simulink model "x2Stage_Rocket"  (R2022b)
settings: Solver=VariableStepAuto  StartTime=0.0  StopTime=5
model workspace: external: MATLAB File C:\Users\Trenton VerKuilen\OneDrive - lmu.edu\School\Capstone\SimscapeImportFiles\x2Stage_Rocket_DataFile.m (data not in the file)
undefined symbols (not defined in the file or in its folder): F, MIL, Moderate, sigbuilder_block, smiData, X, Y, Z
libraries: sm_lib x543, nesl_utility x11, simulink_extras x3, sharedtransform x2, dspmtrx3 x2, aerolibwind2 x2, mspsensorlib x1, aerolibatmos2 x1
(part 6 of 11)

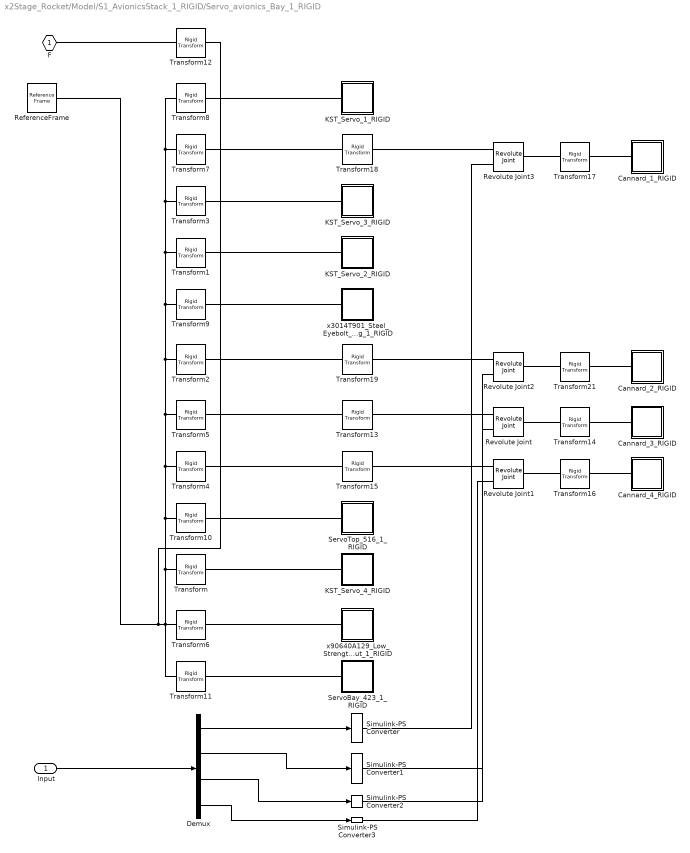
== system x2Stage_Rocket/Model/S1_AvionicsStack_1_RIGID/Servo_avionics_Bay_1_RIGID ==
  Input : Inport
  Cannard_1_RIGID : Subsystem
  Cannard_2_RIGID : Subsystem
  Cannard_3_RIGID : Subsystem
  Cannard_4_RIGID : Subsystem
  Demux : Demux
  KST_Servo_1_RIGID : Subsystem
  KST_Servo_2_RIGID : Subsystem
  KST_Servo_3_RIGID : Subsystem
  KST_Servo_4_RIGID : Subsystem
  ReferenceFrame : sm_lib/Frames and Transforms/Reference Frame
  Revolute Joint{,1..3} (4 alike) : sm_lib/Joints/Revolute Joint  JointMode=Normal  SenseConstraintForce=off  SenseConstraintForceX=off  SenseConstraintForceY=off  SenseConstraintForceZ=off  SenseConstraintTorque=off  SenseConstraintTorqueX=off  SenseConstraintTorqueY=off  SenseConstraintTorqueZ=off  SenseTotalForce=off  SenseTotalForceX=off  SenseTotalForceY=off  SenseTotalForceZ=off  SenseTotalTorque=off  SenseTotalTorqueX=off  SenseTotalTorqueY=off  SenseTotalTorqueZ=off  CompositeWrenchDir=FollowerOnBase  CompositeWrenchFrame=BaseFrame  EquilibriumPosition=0  EquilibriumPositionUnits=deg  SpringStiffness=0  SpringStiffnessUnits=N*m/deg  DampingCoefficient=0  DampingCoefficientUnits=N*m/(deg/s)  TorqueActuationMode=ComputedTorque  MotionActuationMode=InputMotion  SensePosition=off  SenseVelocity=off  SenseAcceleration=off  SenseTorqueForce=off  SenseLowerLimitTorqueForce=off  SenseUpperLimitTorqueForce=off  LowerLimitSpecify=off  LowerLimitBound=-90  LowerLimitBoundUnits=deg  LowerLimitStiffness=1e4  LowerLimitStiffnessUnits=N*m/deg  LowerLimitDamping=10  LowerLimitDampingUnits=N*m/(deg/s)  LowerLimitTransitionRegionWidth=0.1  LowerLimitTransitionRegionWidthUnits=deg  UpperLimitSpecify=off  UpperLimitBound=90  UpperLimitBoundUnits=deg  UpperLimitStiffness=1e4  UpperLimitStiffnessUnits=N*m/deg  UpperLimitDamping=10  UpperLimitDampingUnits=N*m/(deg/s)  UpperLimitTransitionRegionWidth=0.1  UpperLimitTransitionRegionWidthUnits=deg  PositionTargetSpecify=off  PositionTargetPriority=High  PositionTargetValue=0  PositionTargetValueUnits=deg  VelocityTargetSpecify=off  VelocityTargetPriority=High  VelocityTargetValue=0  VelocityTargetValueUnits=deg/s
  ServoBay_423_1_RIGID : Subsystem
  ServoTop_516_1_RIGID : Subsystem
  Simulink-PS Converter{,1..3} (4 alike) : nesl_utility/Simulink-PS Converter  PhysicalDomain=network_engine_domain  SubClassName=ps_input  LeftPortType=input  RightPortType=output  PseudoPeriodic=off  Frequencies=[]  NoiseDistribution=none  NoiseParameters=[]  Unit=1  AffineConversion=off  FilteringAndDerivatives=filter  SimscapeFilterOrder=2  InputFilterTimeConstant=0.001  UdotUserProvided=0
  Transform : sm_lib/Frames and Transforms/Rigid Transform  TranslationMethod=Cartesian  TranslationStandardOffset=0  TranslationLengthUnit=in  TranslationStandardAxis=+Z  TranslationCartesianOffset=smiData.RigidTransform(117).translation  TranslationROffset=0  TranslationROffsetUnits=m  TranslationZOffset=0  TranslationZOffsetUnits=m  TranslationThetaOffset=0  TranslationThetaOffsetUnits=deg  RotationMethod=ArbitraryAxis  RotationAngleUnits=rad  RotationStandardAxis=+Z  RotationAngle=smiData.RigidTransform(117).angle  RotationArbitraryAxis=smiData.RigidTransform(117).axis  FollAlignAxisA=+X  BaseAlignAxisA=+Y  FollAlignAxisB=+Y  BaseAlignAxisB=+Z  RotationSequenceAxes=FollowerAxes  RotationSequence=XYX  RotationSequenceAngles=[0 0 0]  RotationSequenceAnglesUnits=deg  RotationMatrix=[1 0 0; 0 1 0; 0 0 1]  Quaternion=[1 0 0 0]
  Transform1 : sm_lib/Frames and Transforms/Rigid Transform  TranslationMethod=Cartesian  TranslationStandardOffset=0  TranslationLengthUnit=in  TranslationStandardAxis=+Z  TranslationCartesianOffset=smiData.RigidTransform(118).translation  TranslationROffset=0  TranslationROffsetUnits=m  TranslationZOffset=0  TranslationZOffsetUnits=m  TranslationThetaOffset=0  TranslationThetaOffsetUnits=deg  RotationMethod=ArbitraryAxis  RotationAngleUnits=rad  RotationStandardAxis=+Z  RotationAngle=smiData.RigidTransform(118).angle  RotationArbitraryAxis=smiData.RigidTransform(118).axis  FollAlignAxisA=+X  BaseAlignAxisA=+Y  FollAlignAxisB=+Y  BaseAlignAxisB=+Z  RotationSequenceAxes=FollowerAxes  RotationSequence=XYX  RotationSequenceAngles=[0 0 0]  RotationSequenceAnglesUnits=deg  RotationMatrix=[1 0 0; 0 1 0; 0 0 1]  Quaternion=[1 0 0 0]
  Transform10 : sm_lib/Frames and Transforms/Rigid Transform  TranslationMethod=Cartesian  TranslationStandardOffset=0  TranslationLengthUnit=in  TranslationStandardAxis=+Z  TranslationCartesianOffset=smiData.RigidTransform(127).translation  TranslationROffset=0  TranslationROffsetUnits=m  TranslationZOffset=0  TranslationZOffsetUnits=m  TranslationThetaOffset=0  TranslationThetaOffsetUnits=deg  RotationMethod=ArbitraryAxis  RotationAngleUnits=rad  RotationStandardAxis=+Z  RotationAngle=smiData.RigidTransform(127).angle  RotationArbitraryAxis=smiData.RigidTransform(127).axis  FollAlignAxisA=+X  BaseAlignAxisA=+Y  FollAlignAxisB=+Y  BaseAlignAxisB=+Z  RotationSequenceAxes=FollowerAxes  RotationSequence=XYX  RotationSequenceAngles=[0 0 0]  RotationSequenceAnglesUnits=deg  RotationMatrix=[1 0 0; 0 1 0; 0 0 1]  Quaternion=[1 0 0 0]
  Transform11 : sm_lib/Frames and Transforms/Rigid Transform  TranslationMethod=Cartesian  TranslationStandardOffset=0  TranslationLengthUnit=in  TranslationStandardAxis=+Z  TranslationCartesianOffset=smiData.RigidTransform(128).translation  TranslationROffset=0  TranslationROffsetUnits=m  TranslationZOffset=0  TranslationZOffsetUnits=m  TranslationThetaOffset=0  TranslationThetaOffsetUnits=deg  RotationMethod=ArbitraryAxis  RotationAngleUnits=rad  RotationStandardAxis=+Z  RotationAngle=smiData.RigidTransform(128).angle  RotationArbitraryAxis=smiData.RigidTransform(128).axis  FollAlignAxisA=+X  BaseAlignAxisA=+Y  FollAlignAxisB=+Y  BaseAlignAxisB=+Z  RotationSequenceAxes=FollowerAxes  RotationSequence=XYX  RotationSequenceAngles=[0 0 0]  RotationSequenceAnglesUnits=deg  RotationMatrix=[1 0 0; 0 1 0; 0 0 1]  Quaternion=[1 0 0 0]
  Transform12 : sm_lib/Frames and Transforms/Rigid Transform  TranslationMethod=Cartesian  TranslationStandardOffset=0  TranslationLengthUnit=in  TranslationStandardAxis=+Z  TranslationCartesianOffset=smiData.RigidTransform(129).translation  TranslationROffset=0  TranslationROffsetUnits=m  TranslationZOffset=0  TranslationZOffsetUnits=m  TranslationThetaOffset=0  TranslationThetaOffsetUnits=deg  RotationMethod=ArbitraryAxis  RotationAngleUnits=rad  RotationStandardAxis=+Z  RotationAngle=smiData.RigidTransform(129).angle  RotationArbitraryAxis=smiData.RigidTransform(129).axis  FollAlignAxisA=+X  BaseAlignAxisA=+Y  FollAlignAxisB=+Y  BaseAlignAxisB=+Z  RotationSequenceAxes=FollowerAxes  RotationSequence=XYX  RotationSequenceAngles=[0 0 0]  RotationSequenceAnglesUnits=deg  RotationMatrix=[1 0 0; 0 1 0; 0 0 1]  Quaternion=[1 0 0 0]
  Transform{13,16..17,19} (4 alike) : sm_lib/Frames and Transforms/Rigid Transform  TranslationMethod=None  TranslationStandardOffset=0  TranslationLengthUnit=in  TranslationStandardAxis=+Z  TranslationCartesianOffset=smiData.RigidTransform(114).translation  TranslationROffset=0  TranslationROffsetUnits=m  TranslationZOffset=0  TranslationZOffsetUnits=m  TranslationThetaOffset=0  TranslationThetaOffsetUnits=deg  RotationMethod=StandardAxis  RotationAngleUnits=deg  RotationStandardAxis=+Y  RotationAngle=-90  RotationArbitraryAxis=smiData.RigidTransform(114).axis  FollAlignAxisA=+X  BaseAlignAxisA=+Y  FollAlignAxisB=+Y  BaseAlignAxisB=+Z  RotationSequenceAxes=FollowerAxes  RotationSequence=XYX  RotationSequenceAngles=[0 0 0]  RotationSequenceAnglesUnits=deg  RotationMatrix=[1 0 0; 0 1 0; 0 0 1]  Quaternion=[1 0 0 0]
  Transform{14..15,18,21} (4 alike) : sm_lib/Frames and Transforms/Rigid Transform  TranslationMethod=None  TranslationStandardOffset=0  TranslationLengthUnit=in  TranslationStandardAxis=+Z  TranslationCartesianOffset=smiData.RigidTransform(114).translation  TranslationROffset=0  TranslationROffsetUnits=m  TranslationZOffset=0  TranslationZOffsetUnits=m  TranslationThetaOffset=0  TranslationThetaOffsetUnits=deg  RotationMethod=StandardAxis  RotationAngleUnits=deg  RotationStandardAxis=+Y  RotationAngle=90  RotationArbitraryAxis=smiData.RigidTransform(114).axis  FollAlignAxisA=+X  BaseAlignAxisA=+Y  FollAlignAxisB=+Y  BaseAlignAxisB=+Z  RotationSequenceAxes=FollowerAxes  RotationSequence=XYX  RotationSequenceAngles=[0 0 0]  RotationSequenceAnglesUnits=deg  RotationMatrix=[1 0 0; 0 1 0; 0 0 1]  Quaternion=[1 0 0 0]
  Transform2 : sm_lib/Frames and Transforms/Rigid Transform  TranslationMethod=Cartesian  TranslationStandardOffset=0  TranslationLengthUnit=in  TranslationStandardAxis=+Z  TranslationCartesianOffset=smiData.RigidTransform(119).translation  TranslationROffset=0  TranslationROffsetUnits=m  TranslationZOffset=0  TranslationZOffsetUnits=m  TranslationThetaOffset=0  TranslationThetaOffsetUnits=deg  RotationMethod=ArbitraryAxis  RotationAngleUnits=rad  RotationStandardAxis=+Z  RotationAngle=smiData.RigidTransform(119).angle  RotationArbitraryAxis=smiData.RigidTransform(119).axis  FollAlignAxisA=+X  BaseAlignAxisA=+Y  FollAlignAxisB=+Y  BaseAlignAxisB=+Z  RotationSequenceAxes=FollowerAxes  RotationSequence=XYX  RotationSequenceAngles=[0 0 0]  RotationSequenceAnglesUnits=deg  RotationMatrix=[1 0 0; 0 1 0; 0 0 1]  Quaternion=[1 0 0 0]
  Transform3 : sm_lib/Frames and Transforms/Rigid Transform  TranslationMethod=Cartesian  TranslationStandardOffset=0  TranslationLengthUnit=in  TranslationStandardAxis=+Z  TranslationCartesianOffset=smiData.RigidTransform(120).translation  TranslationROffset=0  TranslationROffsetUnits=m  TranslationZOffset=0  TranslationZOffsetUnits=m  TranslationThetaOffset=0  TranslationThetaOffsetUnits=deg  RotationMethod=ArbitraryAxis  RotationAngleUnits=rad  RotationStandardAxis=+Z  RotationAngle=smiData.RigidTransform(120).angle  RotationArbitraryAxis=smiData.RigidTransform(120).axis  FollAlignAxisA=+X  BaseAlignAxisA=+Y  FollAlignAxisB=+Y  BaseAlignAxisB=+Z  RotationSequenceAxes=FollowerAxes  RotationSequence=XYX  RotationSequenceAngles=[0 0 0]  RotationSequenceAnglesUnits=deg  RotationMatrix=[1 0 0; 0 1 0; 0 0 1]  Quaternion=[1 0 0 0]
  Transform4 : sm_lib/Frames and Transforms/Rigid Transform  TranslationMethod=Cartesian  TranslationStandardOffset=0  TranslationLengthUnit=in  TranslationStandardAxis=+Z  TranslationCartesianOffset=smiData.RigidTransform(121).translation  TranslationROffset=0  TranslationROffsetUnits=m  TranslationZOffset=0  TranslationZOffsetUnits=m  TranslationThetaOffset=0  TranslationThetaOffsetUnits=deg  RotationMethod=ArbitraryAxis  RotationAngleUnits=rad  RotationStandardAxis=+Z  RotationAngle=smiData.RigidTransform(121).angle  RotationArbitraryAxis=smiData.RigidTransform(121).axis  FollAlignAxisA=+X  BaseAlignAxisA=+Y  FollAlignAxisB=+Y  BaseAlignAxisB=+Z  RotationSequenceAxes=FollowerAxes  RotationSequence=XYX  RotationSequenceAngles=[0 0 0]  RotationSequenceAnglesUnits=deg  RotationMatrix=[1 0 0; 0 1 0; 0 0 1]  Quaternion=[1 0 0 0]
  Transform5 : sm_lib/Frames and Transforms/Rigid Transform  TranslationMethod=Cartesian  TranslationStandardOffset=0  TranslationLengthUnit=in  TranslationStandardAxis=+Z  TranslationCartesianOffset=smiData.RigidTransform(122).translation  TranslationROffset=0  TranslationROffsetUnits=m  TranslationZOffset=0  TranslationZOffsetUnits=m  TranslationThetaOffset=0  TranslationThetaOffsetUnits=deg  RotationMethod=ArbitraryAxis  RotationAngleUnits=rad  RotationStandardAxis=+Z  RotationAngle=smiData.RigidTransform(122).angle  RotationArbitraryAxis=smiData.RigidTransform(122).axis  FollAlignAxisA=+X  BaseAlignAxisA=+Y  FollAlignAxisB=+Y  BaseAlignAxisB=+Z  RotationSequenceAxes=FollowerAxes  RotationSequence=XYX  RotationSequenceAngles=[0 0 0]  RotationSequenceAnglesUnits=deg  RotationMatrix=[1 0 0; 0 1 0; 0 0 1]  Quaternion=[1 0 0 0]
  Transform6 : sm_lib/Frames and Transforms/Rigid Transform  TranslationMethod=Cartesian  TranslationStandardOffset=0  TranslationLengthUnit=in  TranslationStandardAxis=+Z  TranslationCartesianOffset=smiData.RigidTransform(123).translation  TranslationROffset=0  TranslationROffsetUnits=m  TranslationZOffset=0  TranslationZOffsetUnits=m  TranslationThetaOffset=0  TranslationThetaOffsetUnits=deg  RotationMethod=ArbitraryAxis  RotationAngleUnits=rad  RotationStandardAxis=+Z  RotationAngle=smiData.RigidTransform(123).angle  RotationArbitraryAxis=smiData.RigidTransform(123).axis  FollAlignAxisA=+X  BaseAlignAxisA=+Y  FollAlignAxisB=+Y  BaseAlignAxisB=+Z  RotationSequenceAxes=FollowerAxes  RotationSequence=XYX  RotationSequenceAngles=[0 0 0]  RotationSequenceAnglesUnits=deg  RotationMatrix=[1 0 0; 0 1 0; 0 0 1]  Quaternion=[1 0 0 0]
  Transform7 : sm_lib/Frames and Transforms/Rigid Transform  TranslationMethod=Cartesian  TranslationStandardOffset=0  TranslationLengthUnit=in  TranslationStandardAxis=+Z  TranslationCartesianOffset=smiData.RigidTransform(124).translation  TranslationROffset=0  TranslationROffsetUnits=m  TranslationZOffset=0  TranslationZOffsetUnits=m  TranslationThetaOffset=0  TranslationThetaOffsetUnits=deg  RotationMethod=ArbitraryAxis  RotationAngleUnits=rad  RotationStandardAxis=+Z  RotationAngle=smiData.RigidTransform(124).angle  RotationArbitraryAxis=smiData.RigidTransform(124).axis  FollAlignAxisA=+X  BaseAlignAxisA=+Y  FollAlignAxisB=+Y  BaseAlignAxisB=+Z  RotationSequenceAxes=FollowerAxes  RotationSequence=XYX  RotationSequenceAngles=[0 0 0]  RotationSequenceAnglesUnits=deg  RotationMatrix=[1 0 0; 0 1 0; 0 0 1]  Quaternion=[1 0 0 0]
  Transform8 : sm_lib/Frames and Transforms/Rigid Transform  TranslationMethod=Cartesian  TranslationStandardOffset=0  TranslationLengthUnit=in  TranslationStandardAxis=+Z  TranslationCartesianOffset=smiData.RigidTransform(125).translation  TranslationROffset=0  TranslationROffsetUnits=m  TranslationZOffset=0  TranslationZOffsetUnits=m  TranslationThetaOffset=0  TranslationThetaOffsetUnits=deg  RotationMethod=ArbitraryAxis  RotationAngleUnits=rad  RotationStandardAxis=+Z  RotationAngle=smiData.RigidTransform(125).angle  RotationArbitraryAxis=smiData.RigidTransform(125).axis  FollAlignAxisA=+X  BaseAlignAxisA=+Y  FollAlignAxisB=+Y  BaseAlignAxisB=+Z  RotationSequenceAxes=FollowerAxes  RotationSequence=XYX  RotationSequenceAngles=[0 0 0]  RotationSequenceAnglesUnits=deg  RotationMatrix=[1 0 0; 0 1 0; 0 0 1]  Quaternion=[1 0 0 0]
  Transform9 : sm_lib/Frames and Transforms/Rigid Transform  TranslationMethod=Cartesian  TranslationStandardOffset=0  TranslationLengthUnit=in  TranslationStandardAxis=+Z  TranslationCartesianOffset=smiData.RigidTransform(126).translation  TranslationROffset=0  TranslationROffsetUnits=m  TranslationZOffset=0  TranslationZOffsetUnits=m  TranslationThetaOffset=0  TranslationThetaOffsetUnits=deg  RotationMethod=ArbitraryAxis  RotationAngleUnits=rad  RotationStandardAxis=+Z  RotationAngle=smiData.RigidTransform(126).angle  RotationArbitraryAxis=smiData.RigidTransform(126).axis  FollAlignAxisA=+X  BaseAlignAxisA=+Y  FollAlignAxisB=+Y  BaseAlignAxisB=+Z  RotationSequenceAxes=FollowerAxes  RotationSequence=XYX  RotationSequenceAngles=[0 0 0]  RotationSequenceAnglesUnits=deg  RotationMatrix=[1 0 0; 0 1 0; 0 0 1]  Quaternion=[1 0 0 0]
  x3014T901_Steel_Eyebolt_with_Shoulder_for_Lifting_1_RIGID : Subsystem
  x90640A129_Low_Strength_Steel_Nylon_Insert_Locknut_1_RIGID : Subsystem
  F : PMIOPort  Side=Right
  wires:
  Input/1 -> Demux/1
  Demux/1 -> Simulink-PS Converter/1
  Demux/2 -> Simulink-PS Converter1/1
  Demux/3 -> Simulink-PS Converter2/1
  Demux/4 -> Simulink-PS Converter3/1
  connections:
  F/RConn1 -- Transform12/LConn1
  Revolute Joint1/RConn1 -- Transform16/LConn1
  Transform8/RConn1 -- KST_Servo_1_RIGID/LConn1
  Revolute Joint3/RConn1 -- Transform17/LConn1
  ReferenceFrame/RConn1 -- Transform7/LConn1 -- Transform8/LConn1 -- Transform3/LConn1 -- Transform1/LConn1 -- Transform9/LConn1 -- Transform2/LConn1 -- Transform5/LConn1 -- Transform4/LConn1 -- Transform10/LConn1 -- Transform/LConn1 -- Transform6/LConn1 -- Transform11/LConn1 -- Transform12/RConn1
  Transform3/RConn1 -- KST_Servo_3_RIGID/LConn1
  Transform7/RConn1 -- Transform18/LConn1
  Transform1/RConn1 -- KST_Servo_2_RIGID/LConn1
  Transform9/RConn1 -- x3014T901_Steel_Eyebolt_with_Shoulder_for_Lifting_1_RIGID/LConn1
  Transform2/RConn1 -- Transform19/LConn1
  Transform5/RConn1 -- Transform13/LConn1
  Transform4/RConn1 -- Transform15/LConn1
  Transform10/RConn1 -- ServoTop_516_1_RIGID/LConn1
  Transform/RConn1 -- KST_Servo_4_RIGID/LConn1
  Transform6/RConn1 -- x90640A129_Low_Strength_Steel_Nylon_Insert_Locknut_1_RIGID/LConn1
  Transform11/RConn1 -- ServoBay_423_1_RIGID/LConn1
  Transform19/RConn1 -- Revolute Joint2/LConn1
  Transform18/RConn1 -- Revolute Joint3/LConn1
  Transform13/RConn1 -- Revolute Joint/LConn1
  Transform15/RConn1 -- Revolute Joint1/LConn1
  Simulink-PS Converter/RConn1 -- Revolute Joint3/LConn2
  Simulink-PS Converter1/RConn1 -- Revolute Joint2/LConn2
  Simulink-PS Converter2/RConn1 -- Revolute Joint/LConn2
  Simulink-PS Converter3/RConn1 -- Revolute Joint1/LConn2
  Revolute Joint2/RConn1 -- Transform21/LConn1
  Revolute Joint/RConn1 -- Transform14/LConn1
  Transform17/RConn1 -- Cannard_1_RIGID/LConn1
  Transform21/RConn1 -- Cannard_2_RIGID/LConn1
  Transform14/RConn1 -- Cannard_3_RIGID/LConn1
  Transform16/RConn1 -- Cannard_4_RIGID/LConn1

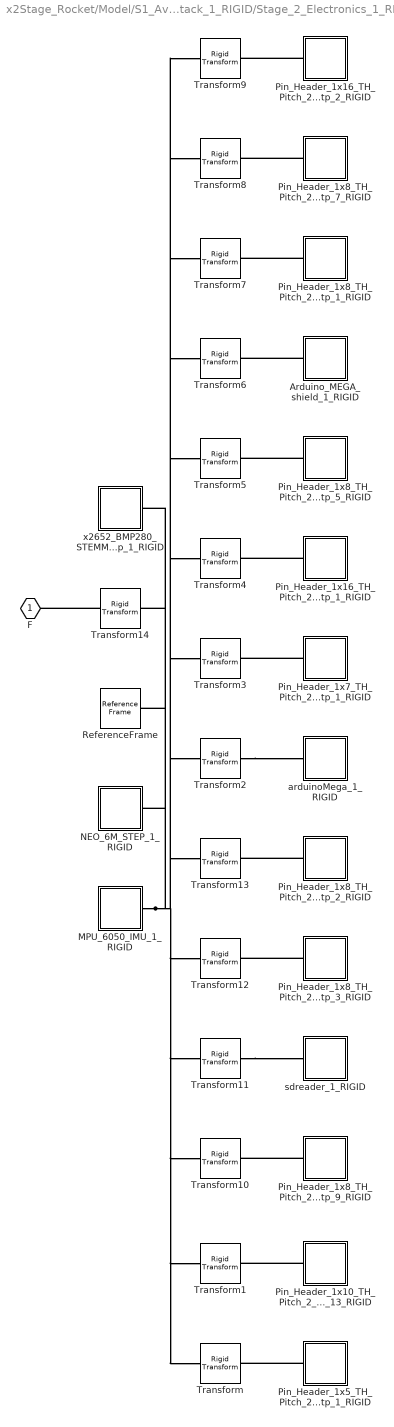
== system x2Stage_Rocket/Model/S1_AvionicsStack_1_RIGID/Stage_2_Electronics_1_RIGID ==
  Arduino_MEGA_shield_1_RIGID : Subsystem
  MPU_6050_IMU_1_RIGID : Subsystem
  NEO_6M_STEP_1_RIGID : Subsystem
  Pin_Header_1x10_TH_Pitch_2_54mm_stp_13_RIGID : Subsystem
  Pin_Header_1x16_TH_Pitch_2_54mm_stp_1_RIGID : Subsystem
  Pin_Header_1x16_TH_Pitch_2_54mm_stp_2_RIGID : Subsystem
  Pin_Header_1x5_TH_Pitch_2_54mm_stp_1_RIGID : Subsystem
  Pin_Header_1x7_TH_Pitch_2_54mm_stp_1_RIGID : Subsystem
  Pin_Header_1x8_TH_Pitch_2_54mm_stp_1_RIGID : Subsystem
  Pin_Header_1x8_TH_Pitch_2_54mm_stp_2_RIGID : Subsystem
  Pin_Header_1x8_TH_Pitch_2_54mm_stp_3_RIGID : Subsystem
  Pin_Header_1x8_TH_Pitch_2_54mm_stp_5_RIGID : Subsystem
  Pin_Header_1x8_TH_Pitch_2_54mm_stp_7_RIGID : Subsystem
  Pin_Header_1x8_TH_Pitch_2_54mm_stp_9_RIGID : Subsystem
  ReferenceFrame : sm_lib/Frames and Transforms/Reference Frame
  Transform : sm_lib/Frames and Transforms/Rigid Transform  TranslationMethod=Cartesian  TranslationStandardOffset=0  TranslationLengthUnit=in  TranslationStandardAxis=+Z  TranslationCartesianOffset=smiData.RigidTransform(77).translation  TranslationROffset=0  TranslationROffsetUnits=m  TranslationZOffset=0  TranslationZOffsetUnits=m  TranslationThetaOffset=0  TranslationThetaOffsetUnits=deg  RotationMethod=ArbitraryAxis  RotationAngleUnits=rad  RotationStandardAxis=+Z  RotationAngle=smiData.RigidTransform(77).angle  RotationArbitraryAxis=smiData.RigidTransform(77).axis  FollAlignAxisA=+X  BaseAlignAxisA=+Y  FollAlignAxisB=+Y  BaseAlignAxisB=+Z  RotationSequenceAxes=FollowerAxes  RotationSequence=XYX  RotationSequenceAngles=[0 0 0]  RotationSequenceAnglesUnits=deg  RotationMatrix=[1 0 0; 0 1 0; 0 0 1]  Quaternion=[1 0 0 0]
  Transform1 : sm_lib/Frames and Transforms/Rigid Transform  TranslationMethod=Cartesian  TranslationStandardOffset=0  TranslationLengthUnit=in  TranslationStandardAxis=+Z  TranslationCartesianOffset=smiData.RigidTransform(78).translation  TranslationROffset=0  TranslationROffsetUnits=m  TranslationZOffset=0  TranslationZOffsetUnits=m  TranslationThetaOffset=0  TranslationThetaOffsetUnits=deg  RotationMethod=ArbitraryAxis  RotationAngleUnits=rad  RotationStandardAxis=+Z  RotationAngle=smiData.RigidTransform(78).angle  RotationArbitraryAxis=smiData.RigidTransform(78).axis  FollAlignAxisA=+X  BaseAlignAxisA=+Y  FollAlignAxisB=+Y  BaseAlignAxisB=+Z  RotationSequenceAxes=FollowerAxes  RotationSequence=XYX  RotationSequenceAngles=[0 0 0]  RotationSequenceAnglesUnits=deg  RotationMatrix=[1 0 0; 0 1 0; 0 0 1]  Quaternion=[1 0 0 0]
  Transform10 : sm_lib/Frames and Transforms/Rigid Transform  TranslationMethod=Cartesian  TranslationStandardOffset=0  TranslationLengthUnit=in  TranslationStandardAxis=+Z  TranslationCartesianOffset=smiData.RigidTransform(87).translation  TranslationROffset=0  TranslationROffsetUnits=m  TranslationZOffset=0  TranslationZOffsetUnits=m  TranslationThetaOffset=0  TranslationThetaOffsetUnits=deg  RotationMethod=ArbitraryAxis  RotationAngleUnits=rad  RotationStandardAxis=+Z  RotationAngle=smiData.RigidTransform(87).angle  RotationArbitraryAxis=smiData.RigidTransform(87).axis  FollAlignAxisA=+X  BaseAlignAxisA=+Y  FollAlignAxisB=+Y  BaseAlignAxisB=+Z  RotationSequenceAxes=FollowerAxes  RotationSequence=XYX  RotationSequenceAngles=[0 0 0]  RotationSequenceAnglesUnits=deg  RotationMatrix=[1 0 0; 0 1 0; 0 0 1]  Quaternion=[1 0 0 0]
  Transform11 : sm_lib/Frames and Transforms/Rigid Transform  TranslationMethod=Cartesian  TranslationStandardOffset=0  TranslationLengthUnit=in  TranslationStandardAxis=+Z  TranslationCartesianOffset=smiData.RigidTransform(88).translation  TranslationROffset=0  TranslationROffsetUnits=m  TranslationZOffset=0  TranslationZOffsetUnits=m  TranslationThetaOffset=0  TranslationThetaOffsetUnits=deg  RotationMethod=ArbitraryAxis  RotationAngleUnits=rad  RotationStandardAxis=+Z  RotationAngle=smiData.RigidTransform(88).angle  RotationArbitraryAxis=smiData.RigidTransform(88).axis  FollAlignAxisA=+X  BaseAlignAxisA=+Y  FollAlignAxisB=+Y  BaseAlignAxisB=+Z  RotationSequenceAxes=FollowerAxes  RotationSequence=XYX  RotationSequenceAngles=[0 0 0]  RotationSequenceAnglesUnits=deg  RotationMatrix=[1 0 0; 0 1 0; 0 0 1]  Quaternion=[1 0 0 0]
  Transform12 : sm_lib/Frames and Transforms/Rigid Transform  TranslationMethod=Cartesian  TranslationStandardOffset=0  TranslationLengthUnit=in  TranslationStandardAxis=+Z  TranslationCartesianOffset=smiData.RigidTransform(89).translation  TranslationROffset=0  TranslationROffsetUnits=m  TranslationZOffset=0  TranslationZOffsetUnits=m  TranslationThetaOffset=0  TranslationThetaOffsetUnits=deg  RotationMethod=ArbitraryAxis  RotationAngleUnits=rad  RotationStandardAxis=+Z  RotationAngle=smiData.RigidTransform(89).angle  RotationArbitraryAxis=smiData.RigidTransform(89).axis  FollAlignAxisA=+X  BaseAlignAxisA=+Y  FollAlignAxisB=+Y  BaseAlignAxisB=+Z  RotationSequenceAxes=FollowerAxes  RotationSequence=XYX  RotationSequenceAngles=[0 0 0]  RotationSequenceAnglesUnits=deg  RotationMatrix=[1 0 0; 0 1 0; 0 0 1]  Quaternion=[1 0 0 0]
  Transform13 : sm_lib/Frames and Transforms/Rigid Transform  TranslationMethod=Cartesian  TranslationStandardOffset=0  TranslationLengthUnit=in  TranslationStandardAxis=+Z  TranslationCartesianOffset=smiData.RigidTransform(106).translation  TranslationROffset=0  TranslationROffsetUnits=m  TranslationZOffset=0  TranslationZOffsetUnits=m  TranslationThetaOffset=0  TranslationThetaOffsetUnits=deg  RotationMethod=ArbitraryAxis  RotationAngleUnits=rad  RotationStandardAxis=+Z  RotationAngle=smiData.RigidTransform(106).angle  RotationArbitraryAxis=smiData.RigidTransform(106).axis  FollAlignAxisA=+X  BaseAlignAxisA=+Y  FollAlignAxisB=+Y  BaseAlignAxisB=+Z  RotationSequenceAxes=FollowerAxes  RotationSequence=XYX  RotationSequenceAngles=[0 0 0]  RotationSequenceAnglesUnits=deg  RotationMatrix=[1 0 0; 0 1 0; 0 0 1]  Quaternion=[1 0 0 0]
  Transform14 : sm_lib/Frames and Transforms/Rigid Transform  TranslationMethod=Cartesian  TranslationStandardOffset=0  TranslationLengthUnit=in  TranslationStandardAxis=+Z  TranslationCartesianOffset=smiData.RigidTransform(111).translation  TranslationROffset=0  TranslationROffsetUnits=m  TranslationZOffset=0  TranslationZOffsetUnits=m  TranslationThetaOffset=0  TranslationThetaOffsetUnits=deg  RotationMethod=ArbitraryAxis  RotationAngleUnits=rad  RotationStandardAxis=+Z  RotationAngle=smiData.RigidTransform(111).angle  RotationArbitraryAxis=smiData.RigidTransform(111).axis  FollAlignAxisA=+X  BaseAlignAxisA=+Y  FollAlignAxisB=+Y  BaseAlignAxisB=+Z  RotationSequenceAxes=FollowerAxes  RotationSequence=XYX  RotationSequenceAngles=[0 0 0]  RotationSequenceAnglesUnits=deg  RotationMatrix=[1 0 0; 0 1 0; 0 0 1]  Quaternion=[1 0 0 0]
  Transform2 : sm_lib/Frames and Transforms/Rigid Transform  TranslationMethod=Cartesian  TranslationStandardOffset=0  TranslationLengthUnit=in  TranslationStandardAxis=+Z  TranslationCartesianOffset=smiData.RigidTransform(79).translation  TranslationROffset=0  TranslationROffsetUnits=m  TranslationZOffset=0  TranslationZOffsetUnits=m  TranslationThetaOffset=0  TranslationThetaOffsetUnits=deg  RotationMethod=ArbitraryAxis  RotationAngleUnits=rad  RotationStandardAxis=+Z  RotationAngle=smiData.RigidTransform(79).angle  RotationArbitraryAxis=smiData.RigidTransform(79).axis  FollAlignAxisA=+X  BaseAlignAxisA=+Y  FollAlignAxisB=+Y  BaseAlignAxisB=+Z  RotationSequenceAxes=FollowerAxes  RotationSequence=XYX  RotationSequenceAngles=[0 0 0]  RotationSequenceAnglesUnits=deg  RotationMatrix=[1 0 0; 0 1 0; 0 0 1]  Quaternion=[1 0 0 0]
  Transform3 : sm_lib/Frames and Transforms/Rigid Transform  TranslationMethod=Cartesian  TranslationStandardOffset=0  TranslationLengthUnit=in  TranslationStandardAxis=+Z  TranslationCartesianOffset=smiData.RigidTransform(80).translation  TranslationROffset=0  TranslationROffsetUnits=m  TranslationZOffset=0  TranslationZOffsetUnits=m  TranslationThetaOffset=0  TranslationThetaOffsetUnits=deg  RotationMethod=ArbitraryAxis  RotationAngleUnits=rad  RotationStandardAxis=+Z  RotationAngle=smiData.RigidTransform(80).angle  RotationArbitraryAxis=smiData.RigidTransform(80).axis  FollAlignAxisA=+X  BaseAlignAxisA=+Y  FollAlignAxisB=+Y  BaseAlignAxisB=+Z  RotationSequenceAxes=FollowerAxes  RotationSequence=XYX  RotationSequenceAngles=[0 0 0]  RotationSequenceAnglesUnits=deg  RotationMatrix=[1 0 0; 0 1 0; 0 0 1]  Quaternion=[1 0 0 0]
  Transform4 : sm_lib/Frames and Transforms/Rigid Transform  TranslationMethod=Cartesian  TranslationStandardOffset=0  TranslationLengthUnit=in  TranslationStandardAxis=+Z  TranslationCartesianOffset=smiData.RigidTransform(81).translation  TranslationROffset=0  TranslationROffsetUnits=m  TranslationZOffset=0  TranslationZOffsetUnits=m  TranslationThetaOffset=0  TranslationThetaOffsetUnits=deg  RotationMethod=ArbitraryAxis  RotationAngleUnits=rad  RotationStandardAxis=+Z  RotationAngle=smiData.RigidTransform(81).angle  RotationArbitraryAxis=smiData.RigidTransform(81).axis  FollAlignAxisA=+X  BaseAlignAxisA=+Y  FollAlignAxisB=+Y  BaseAlignAxisB=+Z  RotationSequenceAxes=FollowerAxes  RotationSequence=XYX  RotationSequenceAngles=[0 0 0]  RotationSequenceAnglesUnits=deg  RotationMatrix=[1 0 0; 0 1 0; 0 0 1]  Quaternion=[1 0 0 0]
  Transform5 : sm_lib/Frames and Transforms/Rigid Transform  TranslationMethod=Cartesian  TranslationStandardOffset=0  TranslationLengthUnit=in  TranslationStandardAxis=+Z  TranslationCartesianOffset=smiData.RigidTransform(82).translation  TranslationROffset=0  TranslationROffsetUnits=m  TranslationZOffset=0  TranslationZOffsetUnits=m  TranslationThetaOffset=0  TranslationThetaOffsetUnits=deg  RotationMethod=ArbitraryAxis  RotationAngleUnits=rad  RotationStandardAxis=+Z  RotationAngle=smiData.RigidTransform(82).angle  RotationArbitraryAxis=smiData.RigidTransform(82).axis  FollAlignAxisA=+X  BaseAlignAxisA=+Y  FollAlignAxisB=+Y  BaseAlignAxisB=+Z  RotationSequenceAxes=FollowerAxes  RotationSequence=XYX  RotationSequenceAngles=[0 0 0]  RotationSequenceAnglesUnits=deg  RotationMatrix=[1 0 0; 0 1 0; 0 0 1]  Quaternion=[1 0 0 0]
  Transform6 : sm_lib/Frames and Transforms/Rigid Transform  TranslationMethod=Cartesian  TranslationStandardOffset=0  TranslationLengthUnit=in  TranslationStandardAxis=+Z  TranslationCartesianOffset=smiData.RigidTransform(83).translation  TranslationROffset=0  TranslationROffsetUnits=m  TranslationZOffset=0  TranslationZOffsetUnits=m  TranslationThetaOffset=0  TranslationThetaOffsetUnits=deg  RotationMethod=ArbitraryAxis  RotationAngleUnits=rad  RotationStandardAxis=+Z  RotationAngle=smiData.RigidTransform(83).angle  RotationArbitraryAxis=smiData.RigidTransform(83).axis  FollAlignAxisA=+X  BaseAlignAxisA=+Y  FollAlignAxisB=+Y  BaseAlignAxisB=+Z  RotationSequenceAxes=FollowerAxes  RotationSequence=XYX  RotationSequenceAngles=[0 0 0]  RotationSequenceAnglesUnits=deg  RotationMatrix=[1 0 0; 0 1 0; 0 0 1]  Quaternion=[1 0 0 0]
  Transform7 : sm_lib/Frames and Transforms/Rigid Transform  TranslationMethod=Cartesian  TranslationStandardOffset=0  TranslationLengthUnit=in  TranslationStandardAxis=+Z  TranslationCartesianOffset=smiData.RigidTransform(84).translation  TranslationROffset=0  TranslationROffsetUnits=m  TranslationZOffset=0  TranslationZOffsetUnits=m  TranslationThetaOffset=0  TranslationThetaOffsetUnits=deg  RotationMethod=ArbitraryAxis  RotationAngleUnits=rad  RotationStandardAxis=+Z  RotationAngle=smiData.RigidTransform(84).angle  RotationArbitraryAxis=smiData.RigidTransform(84).axis  FollAlignAxisA=+X  BaseAlignAxisA=+Y  FollAlignAxisB=+Y  BaseAlignAxisB=+Z  RotationSequenceAxes=FollowerAxes  RotationSequence=XYX  RotationSequenceAngles=[0 0 0]  RotationSequenceAnglesUnits=deg  RotationMatrix=[1 0 0; 0 1 0; 0 0 1]  Quaternion=[1 0 0 0]
  Transform8 : sm_lib/Frames and Transforms/Rigid Transform  TranslationMethod=Cartesian  TranslationStandardOffset=0  TranslationLengthUnit=in  TranslationStandardAxis=+Z  TranslationCartesianOffset=smiData.RigidTransform(85).translation  TranslationROffset=0  TranslationROffsetUnits=m  TranslationZOffset=0  TranslationZOffsetUnits=m  TranslationThetaOffset=0  TranslationThetaOffsetUnits=deg  RotationMethod=ArbitraryAxis  RotationAngleUnits=rad  RotationStandardAxis=+Z  RotationAngle=smiData.RigidTransform(85).angle  RotationArbitraryAxis=smiData.RigidTransform(85).axis  FollAlignAxisA=+X  BaseAlignAxisA=+Y  FollAlignAxisB=+Y  BaseAlignAxisB=+Z  RotationSequenceAxes=FollowerAxes  RotationSequence=XYX  RotationSequenceAngles=[0 0 0]  RotationSequenceAnglesUnits=deg  RotationMatrix=[1 0 0; 0 1 0; 0 0 1]  Quaternion=[1 0 0 0]
  Transform9 : sm_lib/Frames and Transforms/Rigid Transform  TranslationMethod=Cartesian  TranslationStandardOffset=0  TranslationLengthUnit=in  TranslationStandardAxis=+Z  TranslationCartesianOffset=smiData.RigidTransform(86).translation  TranslationROffset=0  TranslationROffsetUnits=m  TranslationZOffset=0  TranslationZOffsetUnits=m  TranslationThetaOffset=0  TranslationThetaOffsetUnits=deg  RotationMethod=ArbitraryAxis  RotationAngleUnits=rad  RotationStandardAxis=+Z  RotationAngle=smiData.RigidTransform(86).angle  RotationArbitraryAxis=smiData.RigidTransform(86).axis  FollAlignAxisA=+X  BaseAlignAxisA=+Y  FollAlignAxisB=+Y  BaseAlignAxisB=+Z  RotationSequenceAxes=FollowerAxes  RotationSequence=XYX  RotationSequenceAngles=[0 0 0]  RotationSequenceAnglesUnits=deg  RotationMatrix=[1 0 0; 0 1 0; 0 0 1]  Quaternion=[1 0 0 0]
  arduinoMega_1_RIGID : Subsystem
  sdreader_1_RIGID : Subsystem
  x2652_BMP280_STEMMA_QT_step_1_RIGID : Subsystem
  F : PMIOPort  Side=Right
  connections:
  Pin_Header_1x5_TH_Pitch_2_54mm_stp_1_RIGID/LConn1 -- Transform/RConn1
  Pin_Header_1x10_TH_Pitch_2_54mm_stp_13_RIGID/LConn1 -- Transform1/RConn1
  Pin_Header_1x8_TH_Pitch_2_54mm_stp_9_RIGID/LConn1 -- Transform10/RConn1
  Transform11/RConn1 -- sdreader_1_RIGID/LConn1
  Pin_Header_1x8_TH_Pitch_2_54mm_stp_3_RIGID/LConn1 -- Transform12/RConn1
  Pin_Header_1x8_TH_Pitch_2_54mm_stp_2_RIGID/LConn1 -- Transform13/RConn1
  MPU_6050_IMU_1_RIGID/RConn1 -- NEO_6M_STEP_1_RIGID/RConn1 -- ReferenceFrame/RConn1 -- Transform/LConn1 -- Transform1/LConn1 -- Transform10/LConn1 -- Transform11/LConn1 -- Transform12/LConn1 -- Transform13/LConn1 -- Transform14/RConn1 -- Transform2/LConn1 -- Transform3/LConn1 -- Transform4/LConn1 -- Transform5/LConn1 -- Transform6/LConn1 -- Transform7/LConn1 -- Transform8/LConn1 -- Transform9/LConn1 -- x2652_BMP280_STEMMA_QT_step_1_RIGID/RConn1
  Transform14/LConn1 -- F/RConn1
  Transform2/RConn1 -- arduinoMega_1_RIGID/LConn1
  Pin_Header_1x7_TH_Pitch_2_54mm_stp_1_RIGID/LConn1 -- Transform3/RConn1
  Pin_Header_1x16_TH_Pitch_2_54mm_stp_1_RIGID/LConn1 -- Transform4/RConn1
  Pin_Header_1x8_TH_Pitch_2_54mm_stp_5_RIGID/LConn1 -- Transform5/RConn1
  Arduino_MEGA_shield_1_RIGID/LConn1 -- Transform6/RConn1
  Pin_Header_1x8_TH_Pitch_2_54mm_stp_1_RIGID/LConn1 -- Transform7/RConn1
  Pin_Header_1x8_TH_Pitch_2_54mm_stp_7_RIGID/LConn1 -- Transform8/RConn1
  Pin_Header_1x16_TH_Pitch_2_54mm_stp_2_RIGID/LConn1 -- Transform9/RConn1

== system x2Stage_Rocket/Model/S1_AvionicsStack_1_RIGID/StagingCoupler_1_RIGID ==
  ReferenceFrame : sm_lib/Frames and Transforms/Reference Frame
  Solid : sm_lib/Body Elements/File Solid  ExtGeomFileName=StagingCoupler_Default_sldprt.STEP  UnitType=FromFile  ExtGeomFileUnits=m  StepReaderType=HEX  ExportConvexHullGeometry=off  InertiaType=Custom  Mass=smiData.Solid(41).mass  MassUnits=kg  CenterOfMass=smiData.Solid(41).CoM  CenterOfMassUnits=cm  MomentsOfInertia=smiData.Solid(41).MoI  MomentsOfInertiaUnits=kg*cm^2  ProductsOfInertia=smiData.Solid(41).PoI  ProductsOfInertiaUnits=kg*cm^2  BasedOnType=DensityFromFile  Density=1000  DensityUnits=kg/m^3  DoExposeReferenceFrame=on  SerializedFrames=<Frames/>  GraphicType=FromGeometry  MarkerShape=Sphere  MarkerSize=10  GraphicVisPropType=SimpleVisualProperties  GraphicDiffuseColor=smiData.Solid(41).color  GraphicSpecularColor=[0.5 0.5 0.5 1.0]  GraphicAmbientColor=[0.15 0.15 0.15 1.0]  GraphicEmissiveColor=[0.0 0.0 0.0 1.0]  GraphicShininess=75  GraphicOpacity=smiData.Solid(41).opacity
  F : PMIOPort  Side=Left
  connections:
  ReferenceFrame/RConn1 -- Solid/RConn1 -- F/RConn1

== system x2Stage_Rocket/Model/S1_AvionicsStack_1_RIGID/x2sLipo_1_RIGID ==
  ReferenceFrame : sm_lib/Frames and Transforms/Reference Frame
  Solid : sm_lib/Body Elements/File Solid  ExtGeomFileName=2sLipo_Default_sldprt.STEP  UnitType=FromFile  ExtGeomFileUnits=m  StepReaderType=HEX  ExportConvexHullGeometry=off  InertiaType=Custom  Mass=smiData.Solid(39).mass  MassUnits=kg  CenterOfMass=smiData.Solid(39).CoM  CenterOfMassUnits=mm  MomentsOfInertia=smiData.Solid(39).MoI  MomentsOfInertiaUnits=kg*mm^2  ProductsOfInertia=smiData.Solid(39).PoI  ProductsOfInertiaUnits=kg*mm^2  BasedOnType=DensityFromFile  Density=1000  DensityUnits=kg/m^3  DoExposeReferenceFrame=on  SerializedFrames=<Frames/>  GraphicType=FromGeometry  MarkerShape=Sphere  MarkerSize=10  GraphicVisPropType=SimpleVisualProperties  GraphicDiffuseColor=smiData.Solid(39).color  GraphicSpecularColor=[0.5 0.5 0.5 1.0]  GraphicAmbientColor=[0.15 0.15 0.15 1.0]  GraphicEmissiveColor=[0.0 0.0 0.0 1.0]  GraphicShininess=75  GraphicOpacity=smiData.Solid(39).opacity
  F : PMIOPort  Side=Left
  connections:
  ReferenceFrame/RConn1 -- Solid/RConn1 -- F/RConn1

== system x2Stage_Rocket/Model/S1_AvionicsStack_1_RIGID/x94435A509_Aluminum_Threaded_Rod_1_1_RIGID ==
  ReferenceFrame : sm_lib/Frames and Transforms/Reference Frame
  Solid : sm_lib/Body Elements/File Solid  ExtGeomFileName=94435A509_Aluminum Threaded Rod (1)_94435A509_sldprt.STEP  UnitType=FromFile  ExtGeomFileUnits=m  StepReaderType=HEX  ExportConvexHullGeometry=off  InertiaType=Custom  Mass=smiData.Solid(10).mass  MassUnits=kg  CenterOfMass=smiData.Solid(10).CoM  CenterOfMassUnits=in  MomentsOfInertia=smiData.Solid(10).MoI  MomentsOfInertiaUnits=kg*in^2  ProductsOfInertia=smiData.Solid(10).PoI  ProductsOfInertiaUnits=kg*in^2  BasedOnType=DensityFromFile  Density=1000  DensityUnits=kg/m^3  DoExposeReferenceFrame=on  SerializedFrames=<Frames/>  GraphicType=FromGeometry  MarkerShape=Sphere  MarkerSize=10  GraphicVisPropType=SimpleVisualProperties  GraphicDiffuseColor=smiData.Solid(10).color  GraphicSpecularColor=[0.5 0.5 0.5 1.0]  GraphicAmbientColor=[0.15 0.15 0.15 1.0]  GraphicEmissiveColor=[0.0 0.0 0.0 1.0]  GraphicShininess=75  GraphicOpacity=smiData.Solid(10).opacity
  F : PMIOPort  Side=Left
  connections:
  ReferenceFrame/RConn1 -- Solid/RConn1 -- F/RConn1

== system x2Stage_Rocket/Model/S1_AvionicsStack_1_RIGID/x94435A509_Aluminum_Threaded_Rod_1_2_RIGID ==
  ReferenceFrame : sm_lib/Frames and Transforms/Reference Frame
  Solid : sm_lib/Body Elements/File Solid  ExtGeomFileName=94435A509_Aluminum Threaded Rod (1)_94435A509_sldprt.STEP  UnitType=FromFile  ExtGeomFileUnits=m  StepReaderType=HEX  ExportConvexHullGeometry=off  InertiaType=Custom  Mass=smiData.Solid(10).mass  MassUnits=kg  CenterOfMass=smiData.Solid(10).CoM  CenterOfMassUnits=in  MomentsOfInertia=smiData.Solid(10).MoI  MomentsOfInertiaUnits=kg*in^2  ProductsOfInertia=smiData.Solid(10).PoI  ProductsOfInertiaUnits=kg*in^2  BasedOnType=DensityFromFile  Density=1000  DensityUnits=kg/m^3  DoExposeReferenceFrame=on  SerializedFrames=<Frames/>  GraphicType=FromGeometry  MarkerShape=Sphere  MarkerSize=10  GraphicVisPropType=SimpleVisualProperties  GraphicDiffuseColor=smiData.Solid(10).color  GraphicSpecularColor=[0.5 0.5 0.5 1.0]  GraphicAmbientColor=[0.15 0.15 0.15 1.0]  GraphicEmissiveColor=[0.0 0.0 0.0 1.0]  GraphicShininess=75  GraphicOpacity=smiData.Solid(10).opacity
  F : PMIOPort  Side=Left
  connections:
  ReferenceFrame/RConn1 -- Solid/RConn1 -- F/RConn1

== system x2Stage_Rocket/Plant/Aerodynamics/Air Properties ==
  Height (m) : Inport
  Display{,1..3} (4 alike) : Display
  Humidity : Constant  Value=10
  ISA Atmosphere Model : aerolibatmos2/ISA Atmosphere Model  custom=off  g=9.80665  gamma=1.4  R=287.0531  L=0.0065  h_trop=11000  h_strat=20000  rho0=1.225  P0=101325  T0=288.15  h0=0
  MATLAB Function : MATLAB Function  TreatAsAtomicUnit=on
  Terminator1 : Terminator
  Density : Outport
  Kin. Visc. : Outport  Port=2
  Speed of Sound : Outport  Port=3
  wires:
  MATLAB Function/2(nu) -> Display1/1, Kin. Visc./1
  MATLAB Function/1(rho) -> Display/1, Density/1
  Humidity/1 -> MATLAB Function/3(h)
  ISA Atmosphere Model/1 -> Display2/1, MATLAB Function/1(t)
  ISA Atmosphere Model/3 -> Display3/1, MATLAB Function/2(p)
  Height (m)/1 -> ISA Atmosphere Model/1
  ISA Atmosphere Model/2 -> Speed of Sound/1
  ISA Atmosphere Model/4 -> Terminator1/1

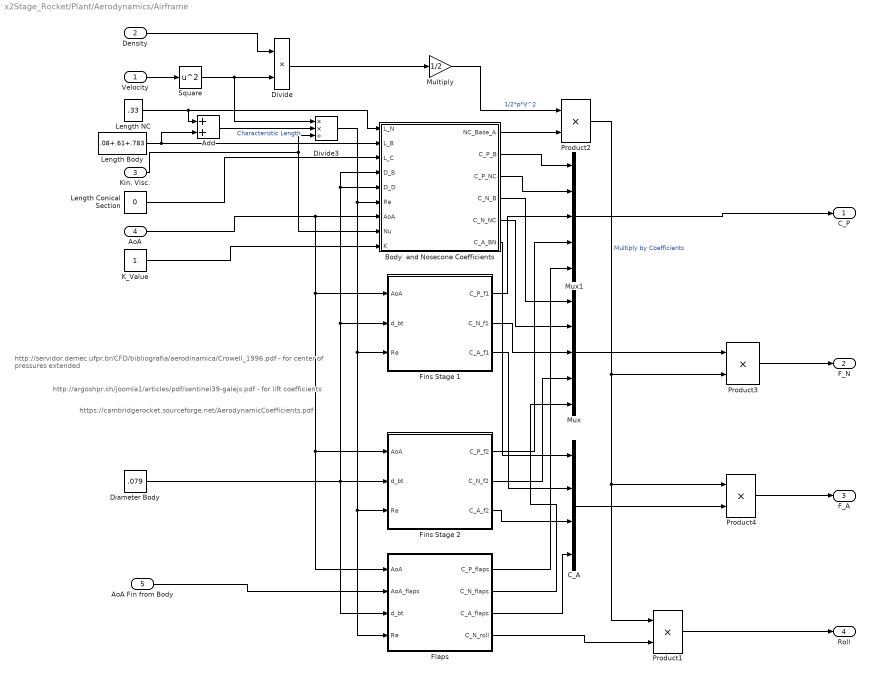
== system x2Stage_Rocket/Plant/Aerodynamics/Airframe ==
  note: https://cambridgerocket.sourceforge.net/AerodynamicCoefficients.pdf
  note: http://servidor.demec.ufpr.br/CFD/bibliografia/aerodinamica/Crowell_1996.pdf - for center of pressures extended
  note: http://argoshpr.ch/joomla1/articles/pdf/sentinel39-galejs.pdf - for lift coefficients
  Velocity : Inport
  Density : Inport  Port=2
  Kin. Visc. : Inport  Port=3
  AoA : Inport  Port=4
  AoA Fin from Body : Inport  Port=5
  Add : Sum
  Body  and Nosecone Coefficients : MATLAB Function  TreatAsAtomicUnit=on
  C_A : Mux
  Diameter Body : Constant  Value=.079
  Divide : Product  Inputs=**
  Divide3 : Product  Inputs=**/
  Fins Stage 1 : MATLAB Function  TreatAsAtomicUnit=on
  Fins Stage 2 : MATLAB Function  TreatAsAtomicUnit=on
  Flaps : MATLAB Function  TreatAsAtomicUnit=on
  K_Value : Constant
  Length Body : Constant  Value=.08+.61+.783
  Length Conical Section : Constant  Value=0
  Length NC : Constant  Value=.33
  Multiply : Gain  Gain=1/2
  Mux : Mux  Inputs=5
  Mux1 : Mux  Inputs=5
  Product{1..4} (4 alike) : Product
  Square : Math  Operator=square
  C_P : Outport
  F_N : Outport  Port=2
  F_A : Outport  Port=3
  Roll : Outport  Port=4
  wires:
  Velocity/1 -> Square/1
  Add/1 -> Divide3/2  "Characteristic Length"
  Product2/1 -> Product1/1, Product4/1, Product3/2  "Multiply by Coefficients"
  Length NC/1 -> Add/1, Body  and Nosecone Coefficients/1(L_N)
  Kin. Visc./1 -> Body  and Nosecone Coefficients/8(Nu), Divide3/3
  Length Body/1 -> Add/2, Body  and Nosecone Coefficients/2(L_B)
  Divide/1 -> Multiply/1
  Density/1 -> Divide/1
  AoA/1 -> Flaps/1(AoA), Fins Stage 2/1(AoA), Fins Stage 1/1(AoA), Body  and Nosecone Coefficients/7(AoA)
  Square/1 -> Divide3/1, Divide/2
  Mux/1 -> Product3/1
  Body  and Nosecone Coefficients/4(C_N_B) -> Mux/1
  Length Conical Section/1 -> Body  and Nosecone Coefficients/3(L_C)
  K_Value/1 -> Body  and Nosecone Coefficients/9(K)
  Diameter Body/1 -> Body  and Nosecone Coefficients/5(D_D), Body  and Nosecone Coefficients/4(D_B), Fins Stage 1/2(d_bt), Flaps/3(d_bt), Fins Stage 2/2(d_bt)
  Fins Stage 2/1(C_P_f2) -> Mux1/4
  Divide3/1 -> Flaps/4(Re), Fins Stage 2/3(Re), Fins Stage 1/3(Re), Body  and Nosecone Coefficients/6(Re)
  Flaps/3(C_A_flaps) -> C_A/4
  Multiply/1 -> Product2/1  "1/2*p*V^2"
  Flaps/1(C_P_flaps) -> Mux1/5
  Body  and Nosecone Coefficients/6(C_A_BN) -> C_A/1
  Body  and Nosecone Coefficients/5(C_N_NC) -> Mux/2
  Fins Stage 2/2(C_N_f2) -> Mux/4
  Fins Stage 2/3(C_A_f2) -> C_A/3
  Flaps/2(C_N_flaps) -> Mux/5
  Mux1/1 -> C_P/1
  Product3/1 -> F_N/1
  Product4/1 -> F_A/1
  Fins Stage 1/2(C_N_f1) -> Mux/3
  Fins Stage 1/3(C_A_f1) -> C_A/2
  Body  and Nosecone Coefficients/3(C_P_NC) -> Mux1/2
  Body  and Nosecone Coefficients/2(C_P_B) -> Mux1/1
  Fins Stage 1/1(C_P_f1) -> Mux1/3
  AoA Fin from Body/1 -> Flaps/2(AoA_flaps)
  Flaps/4(C_N_roll) -> Product1/2
  Product1/1 -> Roll/1
  C_A/1 -> Product4/2
  Body  and Nosecone Coefficients/1(NC_Base_A) -> Product2/2

== system x2Stage_Rocket/Plant/Aerodynamics/Center of Gravity ==
  Demux : Demux  Tag=STV Demux  Outputs=1
      settings: DisplayOption=none
  FromWs : FromWorkspace  Tag=STV FromWs  VariableName=tuvar  ZeroCross=off
      SigBuilderData=|
      | common.afterFinalStr = 'Extrapolate'
      | common.sampleTime = '0'
      | dataSet.timeRange = [0 10]
      | dataSet.name = 'Group 1'
      | sbobj.Groups.Name = 'Group 1'
      | sbobj.Groups.Signals.Name = 'Signal 2'
      | sbobj.Groups.Signals.XData = [0 0.01 0.02 0.03 0.04 0.05 0.06 0.07 0.08 0.09 0.1 0.11 0.12 0.13 0.14 0.15 0.16 0.17 0.18 0.19 0.2 0.21 0.22 0.23 0.24 0.25 0.26 0.27 0.28 0.29 0.3 0.31 0.32 0.33 0.34 0.35 0.36 0.37 0.38 0.39 0.4 0.41 0.42 0.43 0.44 0.455 0.4775 0.51125 0.56125 0.61125 0.66125 0.71125 0.76125 0.81125 0.86125 0.91125 0.95226 0.98929 1.029 1.0781 1.1281 1.1781 1.2281 1.2662 1.3014 1.342 1.392 1.442 1.492 1.5386 1.5886 1.6386 1.6886 1.7386 1.7886 1.8386 1.8886 1.9386 1.9886 2.0386 2.0886 2.1386 2.1886 2.2386 2.2886 2.3386 2.3886 2.4386 2.4886 2.5386 2.5886 2.6386 2.6886 2.7386 2.7886 2.8386 2.8886 10]
      | sbobj.Groups.Signals.YData = [103.89 103.89 103.86 103.83 103.81 103.78 103.76 103.73 103.71 103.69 103.66 103.64 103.61 103.59 103.56 103.54 103.51 103.49 103.47 103.44 103.42 103.39 103.37 103.34 103.32 103.29 103.27 103.24 103.22 103.19 103.17 103.14 103.12 103.09 103.07 103.04 103.02 103 102.97 102.94 102.92 102.89 102.87 102.84 102.82 102.79 102.74 102.67 102.56 102.43 102.3 102.18 102.05 101.93 101.8 101.68 101.57 101.47 101.38 101.27 101.15 101.03 100.92 100.82 100.75 100.68 100.6 100.53 100.48 100.44 100.41 100.38 100.37 100.35 100.35 100.34 100.34 100.34 100.34 100.34 100.34 100.34 100.34 100.34 100.34 100.34 100.34 100.34 100.34 100.34 100.34 100.34 100.34 100.34 100.34 100.34 100.34 100.34]
  Signal 2 : Outport  Tag=STV Outport
  wires:
  FromWs/1 -> Demux/1
  Demux/1 -> Signal 2/1

== system x2Stage_Rocket/Plant/Aerodynamics/Signal Builder ==
  Demux : Demux  Tag=STV Demux  Outputs=2
      settings: DisplayOption=none
  FromWs : FromWorkspace  Tag=STV FromWs  VariableName=tuvar  ZeroCross=off
      SigBuilderData=|
      | common.afterFinalStr = 'Extrapolate'
      | common.sampleTime = '0'
      | dataSet.timeRange = [0 10]
      | dataSet.name = 'Group 1'
      | sbobj.Groups.Name = 'Group 1'
      | sbobj.Groups.Signals(1).Name = 'Logitudinal Moment of Inertia'
      | sbobj.Groups.Signals(1).XData = [0 0.01 0.02 0.03 0.04 0.05 0.06 0.07 0.08 0.09 0.1 0.11 0.12 0.13 0.14 0.15 0.16 0.17 0.18 0.19 0.2 0.21 0.22 0.23 0.24 0.25 0.26 0.27 0.28 0.29 0.3 0.31 0.32 0.33 0.34 0.35 0.36 0.37 0.38 0.39 0.4 0.41 0.42 0.43 0.44 0.455 0.4775 0.51125 0.56125 0.61125 0.66125 0.71125 0.76125 0.81125 0.86125 0.91125 0.95226 0.98929 1.029 1.0781 1.1281 1.1781 1.2281 1.2662 1.3014 1.342 1.392 1.442 1.492 1.5386 1.5886 1.6386 1.6886 1.7386 1.7886 1.8386 1.8886 1.9386 1.9886 2.0386 2.0886 2.1386 2.1886 2.2386 2.2886 2.3386 2.3886 2.4386 2.4886 2.5386 2.5886 2.6386 2.6886 2.7386 2.7886 2.8386 2.8886 10]
      | sbobj.Groups.Signals(1).YData = [0.81527 0.81527 0.81471 0.81406 0.81348 0.81295 0.81241 0.81188 0.81134 0.8108 0.81027 0.80973 0.80919 0.80866 0.80812 0.80758 0.80704 0.8065 0.80596 0.80542 0.80488 0.80434 0.8038 0.80326 0.80272 0.80217 0.80163 0.80109 0.80054 0.8 0.79946 0.79891 0.79836 0.79782 0.79727 0.79673 0.79618 0.79563 0.79508 0.79452 0.79397 0.79342 0.79286 0.79231 0.79175 0.79106 0.79001 0.78844 0.7861 0.7833 0.78048 0.77765 0.77488 0.77216 0.76943 0.76674 0.76432 0.76223 0.76018 0.7578 0.75514 0.75254 0.75002 0.74792 0.74634 0.74477 0.7431 0.74164 0.74043 0.73955 0.7389 0.73835 0.73798 0.73771 0.73753 0.73742 0.73734 0.7373 0.7373 0.7373 0.7373 0.7373 0.7373 0.7373 0.7373 0.7373 0.7373 0.7373 0.7373 0.7373 0.7373 0.7373 0.7373 0.7373 0.7373 0.7373 0.7373 0.7373]
      | sbobj.Groups.Signals(2).Name = 'Rotational Moment of Inertia'
      | sbobj.Groups.Signals(2).XData = [0 0.01 0.02 0.03 0.04 0.05 0.06 0.07 0.08 0.09 0.1 0.11 0.12 0.13 0.14 0.15 0.16 0.17 0.18 0.19 0.2 0.21 0.22 0.23 0.24 0.25 0.26 0.27 0.28 0.29 0.3 0.31 0.32 0.33 0.34 0.35 0.36 0.37 0.38 0.39 0.4 0.41 0.42 0.43 0.44 0.455 0.4775 0.51125 0.56125 0.61125 0.66125 0.71125 0.76125 0.81125 0.86125 0.91125 0.95226 0.98929 1.029 1.0781 1.1281 1.1781 1.2281 1.2662 1.3014 1.342 1.392 1.442 1.492 1.5386 1.5886 1.6386 1.6886 1.7386 1.7886 1.8386 1.8886 1.9386 1.9886 2.0386 2.0886 2.1386 2.1886 2.2386 2.2886 2.3386 2.3886 2.4386 2.4886 2.5386 2.5886 2.6386 2.6886 2.7386 2.7886 2.8386 2.8886 10]
      | sbobj.Groups.Signals(2).YData = [0.010422 0.010422 0.010421 0.010421 0.010421 0.010421 0.010421 0.010421 0.010421 0.01042 0.01042 0.01042 0.01042 0.01042 0.01042 0.01042 0.010419 0.010419 0.010419 0.010419 0.010419 0.010419 0.010419 0.010418 0.010418 0.010418 0.010418 0.010418 0.010418 0.010418 0.010417 0.010417 0.010417 0.010417 0.010417 0.010417 0.010417 0.010416 0.010416 0.010416 0.010416 0.010416 0.010416 0.010416 0.010415 0.010415 0.010415 0.010415 0.010414 0.010413 0.010413 0.010412 0.010411 0.01041 0.01041 0.010409 0.010408 0.010408 0.010407 0.010407 0.010406 0.010406 0.010405 0.010404 0.010404 0.010404 0.010403 0.010403 0.010403 0.010402 0.010402 0.010402 0.010402 0.010402 0.010402 0.010402 0.010402 0.010402 0.010402 0.010402 0.010402 0.010402 0.010402 0.010402 0.010402 0.010402 0.010402 0.010402 0.010402 0.010402 0.010402 0.010402 0.010402 0.010402 0.010402 0.010402 0.010402 0.010402]
  Logitudinal Moment of Inertia : Outport  Tag=STV Outport
  Rotational Moment of Inertia : Outport  Tag=STV Outport  Port=2
  wires:
  Demux/1 -> Logitudinal Moment of Inertia/1
  FromWs/1 -> Demux/1
  Demux/2 -> Rotational Moment of Inertia/1

== system x2Stage_Rocket/Plant/Overall Rocket/Impulse ==
  Demux : Demux  Tag=STV Demux  Outputs=1
      settings: DisplayOption=none
  FromWs : FromWorkspace  Tag=STV FromWs  VariableName=tuvar  ZeroCross=off
      SigBuilderData=|
      | common.afterFinalStr = 'Extrapolate'
      | common.sampleTime = '0'
      | dataSet.timeRange = [0 10]
      | dataSet.name = 'Group 1'
      | sbobj.Groups.Name = 'Group 1'
      | sbobj.Groups.Signals.Name = 'Signal 2'
      | sbobj.Groups.Signals.XData = [0 0.008 0.028 0.36 0.711 0.861 1.121 1.146 1.242 1.349 1.404 1.489 1.602 1.712 1.787 1.892 10]
      | sbobj.Groups.Signals.YData = [0 377.299 241.932 256.333 246.252 233.292 230.411 214.571 211.69 141.127 125.286 72.004 41.762 11.521 12.961 0 0]
  Signal 2 : Outport  Tag=STV Outport
  wires:
  Demux/1 -> Signal 2/1
  FromWs/1 -> Demux/1

== system x2Stage_Rocket/Plant/Overall Rocket/Mass ==
  Demux : Demux  Tag=STV Demux  Outputs=1
      settings: DisplayOption=none
  FromWs : FromWorkspace  Tag=STV FromWs  VariableName=tuvar  ZeroCross=off
      SigBuilderData=|
      | common.afterFinalStr = 'Extrapolate'
      | common.sampleTime = '0'
      | dataSet.timeRange = [0 10]
      | dataSet.name = 'Group 1'
      | sbobj.Groups.Name = 'Group 1'
      | sbobj.Groups.Signals.Name = 'Signal 2'
      | sbobj.Groups.Signals.XData = [0 0.01 0.02 0.03 0.04 0.05 0.06 0.07 0.08 0.09 0.1 0.11 0.12 0.13 0.14 0.15 0.16 0.17 0.18 0.19 0.2 0.21 0.22 0.23 0.24 0.25 0.26 0.27 0.28 0.29 0.3 0.31 0.32 0.33 0.34 0.35 0.36 0.37 0.38 0.39 0.4 0.41 0.42 0.43 0.44 0.455 0.4775 0.51125 0.56125 0.61125 0.66125 0.71125 0.76125 0.81125 0.86125 0.91106 0.9513 0.99131 1.0337 1.0837 1.1337 1.1837 1.2337 1.2765 1.3167 1.3643 1.4143 1.4643 1.5143 1.556 1.606 1.656 1.706 1.756 1.8028 1.8528 1.9028 1.9528 2.0028 2.0528 2.1028 2.1528 2.2028 2.2528 2.3028 2.3528 2.4028 2.4528 2.5028 2.5528 2.6028 2.6528 2.7028 2.7528 2.8028 2.8528 10]
      | sbobj.Groups.Signals.YData = [3464.9 3464.9 3463.5 3461.9 3460.4 3459 3457.7 3456.3 3455 3453.6 3452.3 3450.9 3449.6 3448.2 3446.9 3445.5 3444.2 3442.8 3441.5 3440.1 3438.8 3437.4 3436 3434.7 3433.3 3432 3430.6 3429.3 3427.9 3426.6 3425.2 3423.9 3422.5 3421.2 3419.8 3418.5 3417.1 3415.8 3414.4 3413 3411.7 3410.3 3408.9 3407.6 3406.2 3404.5 3402 3398.1 3392.4 3385.6 3378.8 3372 3365.3 3358.8 3352.3 3345.9 3340.2 3335.2 3330 3324.2 3317.9 3311.9 3306.1 3301.1 3297 3293 3289.2 3286.1 3283.7 3282 3280.6 3279.5 3278.8 3278.3 3278 3277.7 3277.6 3277.5 3277.5 3277.5 3277.5 3277.5 3277.5 3277.5 3277.5 3277.5 3277.5 3277.5 3277.5 3277.5 3277.5 3277.5 3277.5 3277.5 3277.5 3277.5 3277.5]
  Signal 2 : Outport  Tag=STV Outport
  wires:
  FromWs/1 -> Demux/1
  Demux/1 -> Signal 2/1

== system x2Stage_Rocket/Model/AvionicsBay_1_RIGID/Stage_2_Electronics_1_RIGID/Arduino_MEGA_shield_1_RIGID ==
  ReferenceFrame : sm_lib/Frames and Transforms/Reference Frame
  Solid : sm_lib/Body Elements/File Solid  ExtGeomFileName=Arduino MEGA shield_Default_sldprt.STEP  UnitType=FromFile  ExtGeomFileUnits=m  StepReaderType=HEX  ExportConvexHullGeometry=off  InertiaType=Custom  Mass=smiData.Solid(27).mass  MassUnits=kg  CenterOfMass=smiData.Solid(27).CoM  CenterOfMassUnits=mm  MomentsOfInertia=smiData.Solid(27).MoI  MomentsOfInertiaUnits=kg*mm^2  ProductsOfInertia=smiData.Solid(27).PoI  ProductsOfInertiaUnits=kg*mm^2  BasedOnType=DensityFromFile  Density=1000  DensityUnits=kg/m^3  DoExposeReferenceFrame=on  SerializedFrames=<Frames/>  GraphicType=FromGeometry  MarkerShape=Sphere  MarkerSize=10  GraphicVisPropType=SimpleVisualProperties  GraphicDiffuseColor=smiData.Solid(27).color  GraphicSpecularColor=[0.5 0.5 0.5 1.0]  GraphicAmbientColor=[0.15 0.15 0.15 1.0]  GraphicEmissiveColor=[0.0 0.0 0.0 1.0]  GraphicShininess=75  GraphicOpacity=smiData.Solid(27).opacity
  F : PMIOPort  Side=Left
  connections:
  ReferenceFrame/RConn1 -- Solid/RConn1 -- F/RConn1
